simulink model "test_torpedo"  (Simulink 7.6)
settings: Solver=FixedStepDiscrete  StartTime=0.0  StopTime=0  RelTol=1e-3
undefined symbols (not defined in the file or in its folder): gray, Rec, Scale_Forward_B, Scale_Forward_G, Scale_Forward_H, Scale_Forward_R, Scale_Forward_S, Scale_Forward_V, SDTV
libraries: vipsnks x4, vipconversions x3, viptextngfix x1, vipsrcs x1
settings Model: Creator=Thing 1  LastModifiedBy=auvt
settings RTWCC: TargetLang=C++

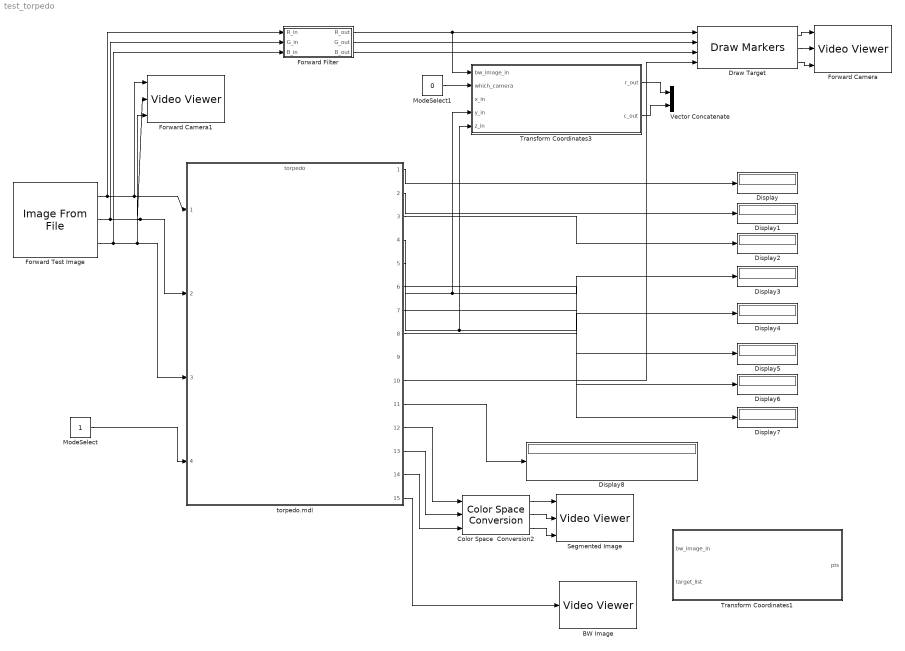
== system test_torpedo ==
  BW Image : vipsnks/Video Viewer  DialogControllerArgs=DataTag1  inputType=Obsolete7b  imagePorts=One multidimensional signal  useColorMap=off  colormapValue=gray(256)  specRange=off  minInputVal=0  maxInputVal=255  FigPos=[1131 861 268 224]  AxisZoom=on  trueSizedOnce=off  OpenAtMdlStart=on
  Color Space  Conversion2 : vipconversions/Color Space  Conversion  conversion=Obsolete  conversionActive=L*a*b* to sR'G'B'  wp_str=D50  rec=Rec. 601 (SDTV)  sys=1125/60/2:1  imagePorts=Separate color signals
  Display{,1..8} (9 alike) : Display
  Draw Target : viptextngfix/Draw Markers  DialogController=vipDDGCreate  DialogControllerArgs=DataTag2  shape=X-mark  size=7  fill=off  fillClrSource=Specify via dialog  display=User-specified value  intensity=200  color=[0 0 0]  opacity=0.6  viewport=Entire image  antialiasing=off  inType=Obsolete  imagePorts=Separate color signals  prodOutputMode=Binary point scaling  prodOutputWordLength=32  prodOutputFracLength=14  memoryMode=Specify word length  memoryWordLength=16  memoryFracLength=15  roundingMode=Floor  overflowMode=off
  Forward Camera : vipsnks/Video Viewer  DialogControllerArgs=DataTag4  inputType=Obsolete7b  imagePorts=Separate color signals  useColorMap=off  colormapValue=gray(256)  specRange=off  minInputVal=0  maxInputVal=255  FigPos=[1096 387 268 224]  AxisZoom=on  trueSizedOnce=off  OpenAtMdlStart=on
  Forward Camera1 : vipsnks/Video Viewer  DialogControllerArgs=DataTag6  inputType=Obsolete7b  imagePorts=Separate color signals  useColorMap=off  colormapValue=gray(256)  specRange=off  minInputVal=0  maxInputVal=255  FigPos=[1096 387 268 224]  AxisZoom=on  trueSizedOnce=off  OpenAtMdlStart=on
  Forward Filter : Subsystem
  Forward Test Image : vipsrcs/Image From File  Tag=vipblks_nd  DialogController=vipDDGCreate  DialogControllerArgs=DataTag7  SystemSampleTime=-1  FileName=/home/auvt/auvc/src/vision/Test_Images/torpedo1.PNG  imagePorts=Separate color signals  Ts=-1  ImageDataType=double  Signed=on  WordLength=16  sdImageDataType=uint(8)  FractionLengthMode=User-defined  FractionLength=15  OutPortLabels=R|G|B
  ModeSelect : Constant  SampleTime=-1
  ModeSelect1 : Constant  Value=0  SampleTime=-1
  Segmented Image : vipsnks/Video Viewer  DialogControllerArgs=DataTag9  inputType=Obsolete7b  imagePorts=Separate color signals  useColorMap=off  colormapValue=gray(256)  specRange=off  minInputVal=0  maxInputVal=255  FigPos=[1082 564 275 212]  AxisZoom=on  trueSizedOnce=off  OpenAtMdlStart=on
  Transform Coordinates1 : Stateflow chart  TreatAsAtomicUnit=on  SystemSampleTime=[1/30 0]
  Transform Coordinates3 : Stateflow chart  TreatAsAtomicUnit=on  SystemSampleTime=[1/30 0]
  Vector Concatenate : Concatenate  Mode=Multidimensional array
  torpedo.mdl : ModelReference  ModelNameDialog=torpedo  SimulationMode=Accelerator  ModelReferenceVersion=1.1062  CopyOfModelName=torpedo
  wires:
  Forward Test Image/1 -> Forward Filter/1(R_in), torpedo.mdl/1, Forward Camera1/1
  Forward Test Image/3 -> Forward Filter/3(B_in), torpedo.mdl/3, Forward Camera1/3
  Draw Target/2 -> Forward Camera/2
  Draw Target/1 -> Forward Camera/1
  Draw Target/3 -> Forward Camera/3
  Forward Filter/1(R_out) -> Draw Target/1, Transform Coordinates3/1(bw_image_in)
  Forward Filter/2(G_out) -> Draw Target/2
  Forward Filter/3(B_out) -> Draw Target/3
  Forward Test Image/2 -> Forward Filter/2(G_in), torpedo.mdl/2, Forward Camera1/2
  ModeSelect1/1 -> Transform Coordinates3/2(which_camera)
  Transform Coordinates3/1(r_out) -> Vector Concatenate/1
  ModeSelect/1 -> torpedo.mdl/4
  torpedo.mdl/1 -> Display/1
  torpedo.mdl/2 -> Display1/1
  torpedo.mdl/3 -> Display2/1
  torpedo.mdl/4 -> Display3/1, Transform Coordinates3/4(y_in)
  torpedo.mdl/5 -> Display4/1, Transform Coordinates3/5(z_in)
  torpedo.mdl/6 -> Display5/1
  torpedo.mdl/7 -> Display6/1
  torpedo.mdl/8 -> Display7/1
  Transform Coordinates3/2(c_out) -> Vector Concatenate/2
  torpedo.mdl/11 -> Display8/1
  torpedo.mdl/10 -> Draw Target/4
  Color Space  Conversion2/1 -> Segmented Image/1
  Color Space  Conversion2/2 -> Segmented Image/2
  Color Space  Conversion2/3 -> Segmented Image/3
  torpedo.mdl/12 -> Color Space  Conversion2/1
  torpedo.mdl/13 -> Color Space  Conversion2/2
  torpedo.mdl/14 -> Color Space  Conversion2/3
  torpedo.mdl/15 -> BW Image/1

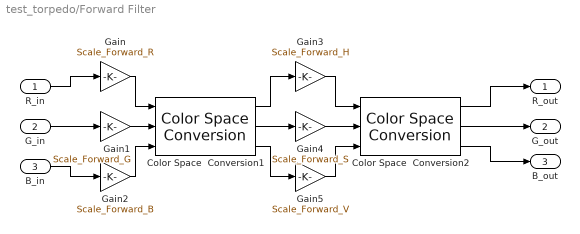
== system test_torpedo/Forward Filter ==
  R_in : Inport  PortDimensions=Forward_Camera_Dimensions
  G_in : Inport  Port=2  PortDimensions=Forward_Camera_Dimensions
  B_in : Inport  Port=3  PortDimensions=Forward_Camera_Dimensions
  Color Space  Conversion1 : vipconversions/Color Space  Conversion  conversion=Obsolete  conversionActive=R'G'B' to HSV  wp_str=D50  rec=Rec. 601 (SDTV)  sys=1125/60/2:1  imagePorts=Separate color signals
  Color Space  Conversion2 : vipconversions/Color Space  Conversion  conversion=Obsolete  conversionActive=HSV to R'G'B'  wp_str=D50  rec=Rec. 601 (SDTV)  sys=1125/60/2:1  imagePorts=Separate color signals
  Gain : Gain  Gain=Scale_Forward_R
  Gain1 : Gain  Gain=Scale_Forward_G
  Gain2 : Gain  Gain=Scale_Forward_B
  Gain3 : Gain  Gain=Scale_Forward_H
  Gain4 : Gain  Gain=Scale_Forward_S
  Gain5 : Gain  Gain=Scale_Forward_V
  R_out : Outport  OutDataTypeStr=double
  G_out : Outport  Port=2  OutDataTypeStr=double
  B_out : Outport  Port=3  OutDataTypeStr=double
  wires:
  R_in/1 -> Gain/1
  G_in/1 -> Gain1/1
  B_in/1 -> Gain2/1
  Gain/1 -> Color Space  Conversion1/1
  Gain1/1 -> Color Space  Conversion1/2
  Gain2/1 -> Color Space  Conversion1/3
  Color Space  Conversion1/1 -> Gain3/1
  Color Space  Conversion1/2 -> Gain4/1
  Color Space  Conversion1/3 -> Gain5/1
  Gain3/1 -> Color Space  Conversion2/1
  Gain4/1 -> Color Space  Conversion2/2
  Gain5/1 -> Color Space  Conversion2/3
  Color Space  Conversion2/1 -> R_out/1
  Color Space  Conversion2/2 -> G_out/1
  Color Space  Conversion2/3 -> B_out/1

== matlab function Transform Coordinates3 ==
  data: bw_image_in input double; which_camera input double; x_in input double; y_in input double; r_out output double; c_out output double; z_in input double
function [r_out, c_out] = transform_G2L(bw_image_in, which_camera, x_in, y_in, z_in)
% This function, "transform Global to Local coordinates," transforms
%   global coordinates that are sent to the controller into local
%   coordinates that can be displayed over images.
%
% 5-29-11
%
% Input
%   x_in, y_in, z_in = vectors of points in global (vehicle-centered)
%     coordinate system
%   bw_image_in = a 2-D array of pixel values (used only to extract image
%     size)
%   which_camera = selects which camera for relative coordinates
%                = 0 -> Forward camera
%                = 1 -> Down camera
%
% Output
%   r_out, c_out = row, column pairs in local coordinate system

[rows, cols] = size(bw_image_in);
if( which_camera == 0 )
    r_out = z_in + floor(rows/2);
    c_out = y_in + floor(cols/2);
else
    r_out = floor(rows/2) - x_in;
    c_out = y_in + floor(cols/2);
end

return

== matlab function Transform Coordinates1 ==
  data: bw_image_in input double; target_list input double; pts output double
function pts  = display_target_list(bw_image_in, target_list)
[rows, cols] = size(bw_image_in);
pts = zeros(2, 50);
%{
for t = 1:3
    pts(1,t) = target_list(1,t);
    pts(
    %}
return
